simulink model "LineFaultModel_online_detection_location_class_by_ann"  (R2022b)
settings: Solver=FixedStepAuto  StartTime=0.0  StopTime=0.2  RelTol=1e-3  EnableMultiTasking=on
undefined symbols (not defined in the file or in its folder): D1, Delta
libraries: neural x29, spsThreePhaseVIMeasurementLib x3, spsRMSLib x2, spsThreePhaseSourceLib x2, spsSequenceAnalyzerLib x2, spsThreePhasePISectionLineLib x2, spsThreePhaseTransformerTwoWindingsLib x1, simulink x1, spsThreePhaseParallelRLCLoadLib x1, spsThreePhaseFaultLib x1, sps_lib x1
(part 2 of 2)

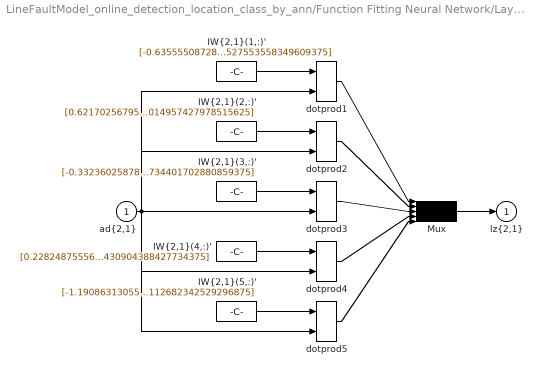
== system LineFaultModel_online_detection_location_class_by_ann/Function Fitting Neural Network/Layer 2/LW{2,1} ==
  "ad{2,1}" : Inport  PortDimensions=20
      mask Display: e = 0.06;c1 = [120 230 180]/255;c2 = ([120 230 180]+0)/(256+128);c3 = ([120 230 180]+128)/(256+128);patch([0 1 1 0],[0 0 1 1],c1);patch([0 1 1 1-e 1-e 0+e],[0 0 1 1-e 0+e 0+e],c2);patch([0 0 1 1-e 0+e 0+e],[0 1 1 1-e 1-e 0+e],c3);plot([0 1 1 0 0],[0 0 1 1 0]);
  "IW{2,1}(1,:)'" : Constant  Value=[-0.6355550872854094368591404418111778795719146728515625;0.454280348367591180203106659973855130374431610107421875;0.05001752503606009259140563472101348452270030975341796875;-0.044941700804318966688821745947279850952327251434326171875;-0.129899733610959022822584074674523435533046722412109375;0.0255621996761338822479192600667374790646135807037353515625;0.2410327286829592463579530203787726350128650665283203125;0.1155393338003729841734212868686881847679615020751953125;0.55685654005267426480685344358789734542369842529296875;0.1666617932670526325278359536241623573005199432373046875;-0.327393491644324796663312326927552931010723114013671875;-0.349758534244095919962802554437075741589069366455078125;0.73732913148962475613501510451897047460079193115234375;-0.66425257085593847339310968891368247568607330322265625;-0.156600182926470432587251480072154663503170013427734375;-0.215478988577362640111090286154649220407009124755859375;-0.72863067397588110463146904294262640178203582763671875;-0.85623858911348194045132231622119434177875518798828125;-0.170606357486681681212559169580345042049884796142578125;0.060226633338919109694753473149830824695527553558349609375]
      mask Display: e = 0.06;c1 = [120 150 230]/255;c2 = ([120 150 230]+0)/383;c3 = ([120 150 230]+128)/383;patch([0 1 1 0],[0 0 1 1],c1);patch([0 1 1 1-e 1-e 0+e],[0 0 1 1-e 0+e 0+e],c2);patch([0 0 1 1-e 0+e 0+e],[0 1 1 1-e 1-e 0+e],c3);plot([0 1 1 0 0],[0 0 1 1 0]);disp('weights');
  "IW{2,1}(2,:)'" : Constant  Value=[0.62170256795246581216218828558339737355709075927734375;-0.31133503032995790693604476473410613834857940673828125;-0.5055805094175733760408775196992792189121246337890625;-0.037152597765622262515616824885000823996961116790771484375;-0.2065036821430944746769142739140079356729984283447265625;0.68403826133888345761846494497149251401424407958984375;0.53573173877781787854956974115339107811450958251953125;0.07126822895831740056760139623293071053922176361083984375;0.470252060464070087419941046391613781452178955078125;-0.210128185115308230290764868186670355498790740966796875;-0.3539266381530044025538472851621918380260467529296875;-0.7231592351147939634614658643840812146663665771484375;0.59220766329617668954909959211363457143306732177734375;0.151791367181647596229510099874460138380527496337890625;-0.031329904272530829933973706147298798896372318267822265625;-0.166945149470736853292152090944000519812107086181640625;0.03903318943470691915198500510086887516081333160400390625;0.055307842010659934162131179391508339904248714447021484375;0.1879351840230618908567095104444888420403003692626953125;0.249295127135879202029400403262116014957427978515625]
      mask Display: e = 0.06;c1 = [120 150 230]/255;c2 = ([120 150 230]+0)/383;c3 = ([120 150 230]+128)/383;patch([0 1 1 0],[0 0 1 1],c1);patch([0 1 1 1-e 1-e 0+e],[0 0 1 1-e 0+e 0+e],c2);patch([0 0 1 1-e 0+e 0+e],[0 1 1 1-e 1-e 0+e],c3);plot([0 1 1 0 0],[0 0 1 1 0]);disp('weights');
  "IW{2,1}(3,:)'" : Constant  Value=[-0.33236025878526487264963407142204232513904571533203125;0.1482617692265812137097924505724222399294376373291015625;-0.55689264853705378044423923711292445659637451171875;0.401442662817064477298600877475109882652759552001953125;0.433875861945531682284382668512989766895771026611328125;-0.1490040069660174826271514803011086769402027130126953125;-0.1607081134209118189470899551452021114528179168701171875;-0.313678056286047446388209891665610484778881072998046875;-0.1330184266684643901168527690970222465693950653076171875;0.87180699842347830763600313730421476066112518310546875;-0.1936204335795219666493949262076057493686676025390625;0.392656926974071784908204563180333934724330902099609375;-0.333656385257076804062847941168001852929592132568359375;0.456026294288772504614826175384223461151123046875;0.57925766625745300775207624610629864037036895751953125;-0.015095716546288211190596229016591678373515605926513671875;0.25156499605062532243238138107699342072010040283203125;-0.164034899653683563514050547382794320583343505859375;-0.5524347416902484209089152500382624566555023193359375;-0.0179830597078222374773925906765725812874734401702880859375]
      mask Display: e = 0.06;c1 = [120 150 230]/255;c2 = ([120 150 230]+0)/383;c3 = ([120 150 230]+128)/383;patch([0 1 1 0],[0 0 1 1],c1);patch([0 1 1 1-e 1-e 0+e],[0 0 1 1-e 0+e 0+e],c2);patch([0 0 1 1-e 0+e 0+e],[0 1 1 1-e 1-e 0+e],c3);plot([0 1 1 0 0],[0 0 1 1 0]);disp('weights');
  "IW{2,1}(4,:)'" : Constant  Value=[0.22824875556678858590231584457796998322010040283203125;-0.351588325346228913748092281821300275623798370361328125;-0.1065433401634824084336372607140219770371913909912109375;-0.07176145605508620073376135906073614023625850677490234375;-0.1647758402428784185733690037523047067224979400634765625;-0.1323938699440107835680890957519295625388622283935546875;-0.25789976224759814105169652975746430456638336181640625;-0.278888504627190225715338556256028823554515838623046875;-0.449204434393933926816799839798477478325366973876953125;-0.285664787820202048518325455006561242043972015380859375;-1.2283947739745817440137898302054964005947113037109375;-0.0772196103313375348253799757003434933722019195556640625;-0.288590159666089363099672482348978519439697265625;0.30062517668017252336909450605162419378757476806640625;-0.1062715914805141270704780254163779318332672119140625;-0.467806400431584723520472834934480488300323486328125;-0.25592934195709859945822017834871076047420501708984375;-0.375236352476599976935034419511794112622737884521484375;-0.410267194148465075276277502780430950224399566650390625;0.85534678031987476654052215963019989430904388427734375]
      mask Display: e = 0.06;c1 = [120 150 230]/255;c2 = ([120 150 230]+0)/383;c3 = ([120 150 230]+128)/383;patch([0 1 1 0],[0 0 1 1],c1);patch([0 1 1 1-e 1-e 0+e],[0 0 1 1-e 0+e 0+e],c2);patch([0 0 1 1-e 0+e 0+e],[0 1 1 1-e 1-e 0+e],c3);plot([0 1 1 0 0],[0 0 1 1 0]);disp('weights');
  "IW{2,1}(5,:)'" : Constant  Value=[-1.19086313055029879848234486416913568973541259765625;-2.00874996530946514639026645454578101634979248046875;2.38353545243033604350557652651332318782806396484375;1.267595673487491136910421118955127894878387451171875;-3.583628653166014199626943081966601312160491943359375;1.1418769558660806229255513244424946606159210205078125;2.057223905859620227687400983995757997035980224609375;-1.7840617857415157487821488757617771625518798828125;-4.7159738144487359789991387515328824520111083984375;4.8879843384569152675567238475196063518524169921875;-3.3864943095206019307852329802699387073516845703125;3.415722562325356204127047021756879985332489013671875;-4.91079674214851191749175995937548577785491943359375;1.3604347008910815386428794226958416402339935302734375;-5.4461517282579539056541761965490877628326416015625;3.135480520453735042707421598606742918491363525390625;2.18213149891216229292467687628231942653656005859375;-4.19956576822003579962938601966015994548797607421875;3.317890425081923666539296391420066356658935546875;-3.61569861614154586249014755594544112682342529296875]
      mask Display: e = 0.06;c1 = [120 150 230]/255;c2 = ([120 150 230]+0)/383;c3 = ([120 150 230]+128)/383;patch([0 1 1 0],[0 0 1 1],c1);patch([0 1 1 1-e 1-e 0+e],[0 0 1 1-e 0+e 0+e],c2);patch([0 0 1 1-e 0+e 0+e],[0 1 1 1-e 1-e 0+e],c3);plot([0 1 1 0 0],[0 0 1 1 0]);disp('weights');
  Mux : Mux  Inputs=5
      mask Display: e = 0.06;c1 = [120 150 230]/255;c2 = ([120 150 230]+0)/383;c3 = ([120 150 230]+128)/383;patch([0 1 1 0],[0 0 1 1],c1);patch([0 1 1 1-e 1-e 0+e],[0 0 1 1-e 0+e 0+e],c2);patch([0 0 1 1-e 0+e 0+e],[0 1 1 1-e 1-e 0+e],c3);plot([0 1 1 0 0],[0 0 1 1 0]);disp('Mux');
  dotprod{1..5} (5 alike) : neural/Weight Functions/dotprod
  "lz{2,1}" : Outport
      mask Display: e = 0.06;c1 = [120 230 180]/255;c2 = ([120 230 180]+0)/(256+128);c3 = ([120 230 180]+128)/(256+128);patch([0 1 1 0],[0 0 1 1],c1);patch([0 1 1 1-e 1-e 0+e],[0 0 1 1-e 0+e 0+e],c2);patch([0 0 1 1-e 0+e 0+e],[0 1 1 1-e 1-e 0+e],c3);plot([0 1 1 0 0],[0 0 1 1 0]);
  wires:
  Mux/1 -> "lz{2,1}"/1
  dotprod5/1 -> Mux/5
  "IW{2,1}(5,:)'"/1 -> dotprod5/1
  dotprod4/1 -> Mux/4
  "IW{2,1}(4,:)'"/1 -> dotprod4/1
  dotprod3/1 -> Mux/3
  "IW{2,1}(3,:)'"/1 -> dotprod3/1
  dotprod2/1 -> Mux/2
  "IW{2,1}(2,:)'"/1 -> dotprod2/1
  dotprod1/1 -> Mux/1
  "ad{2,1}"/1 -> dotprod5/2, dotprod4/2, dotprod3/2, dotprod2/2, dotprod1/2
  "IW{2,1}(1,:)'"/1 -> dotprod1/1
